simulink model "Laba2_2"  (R2022a)
settings: Solver=VariableStepAuto  StartTime=0.0  StopTime=10.0  RelTol=1e-3
settings Model: Creator=38098  LastModifiedBy=38098

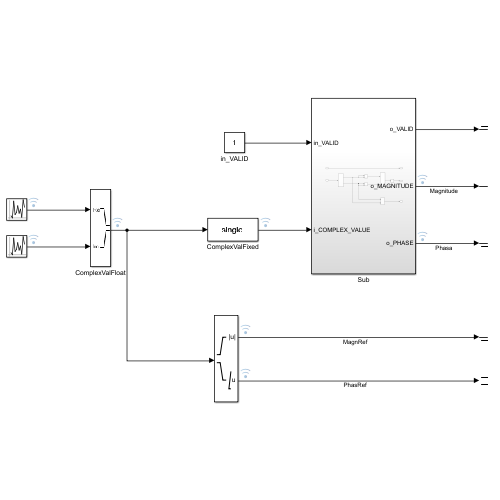
[thumbnail: Simulink's stored preview of the top-level diagram]
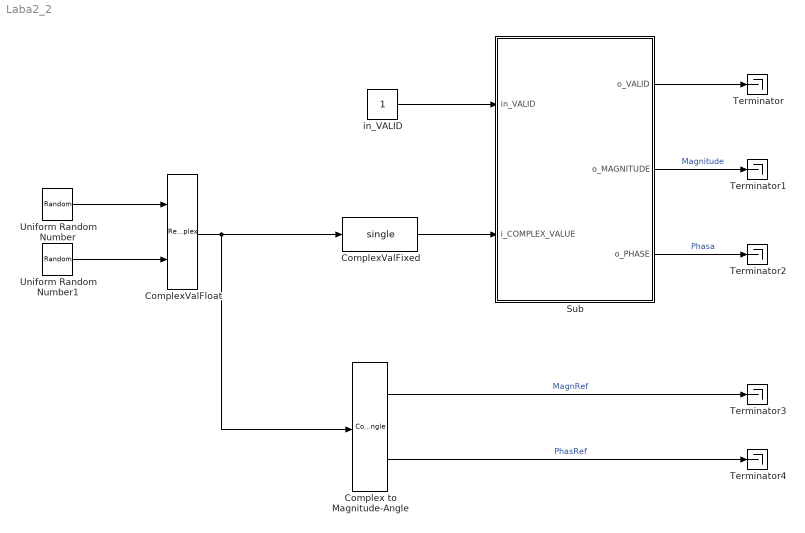
== system Laba2_2 ==
  Complex to Magnitude-Angle : ComplexToMagnitudeAngle
  ComplexValFixed : DataTypeConversion  OutDataTypeStr=single  RndMeth=Round  SaturateOnIntegerOverflow=off
  ComplexValFloat : RealImagToComplex
  Sub : Subsystem
  Terminator{,1..4} (5 alike) : Terminator
  Uniform Random Number : UniformRandomNumber  Minimum=0  Maximum=2 ^(22)-1  Seed=22  SampleTime=1
  Uniform Random Number1 : UniformRandomNumber  Minimum=0  Maximum=2 ^(22)-1  Seed=23  SampleTime=1
  in_VALID : Constant  OutDataTypeStr=boolean  SampleTime=1
  wires:
  Complex to Magnitude-Angle/1 -> Terminator3/1  "MagnRef"
  Sub/1(o_VALID) -> Terminator/1
  Uniform Random Number/1 -> ComplexValFloat/1
  Complex to Magnitude-Angle/2 -> Terminator4/1  "PhasRef"
  in_VALID/1 -> Sub/1(in_VALID)
  Sub/2(o_MAGNITUDE) -> Terminator1/1  "Magnitude"
  ComplexValFloat/1 -> Complex to Magnitude-Angle/1, ComplexValFixed/1
  Uniform Random Number1/1 -> ComplexValFloat/2
  ComplexValFixed/1 -> Sub/2(i_COMPLEX_VALUE)
  Sub/3(o_PHASE) -> Terminator2/1  "Phasa"

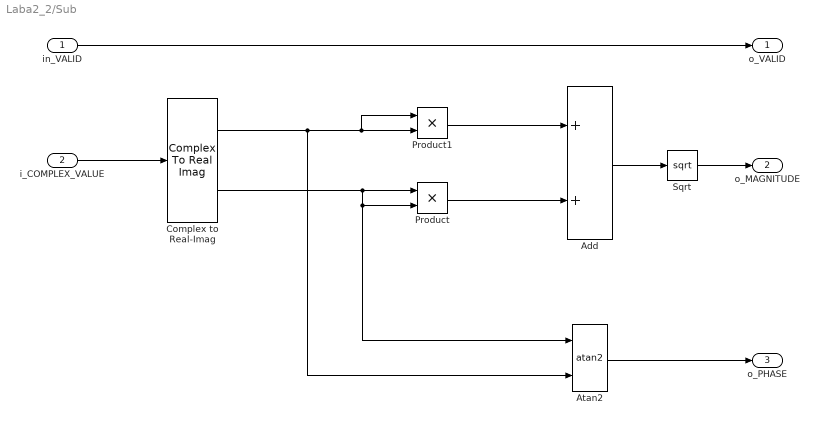
== system Laba2_2/Sub ==
  in_VALID : Inport  OutDataTypeStr=boolean
  i_COMPLEX_VALUE : Inport  Port=2
  Add : Sum
  Atan2 : Trigonometry  Operator=atan2  ApproximationMethod=CORDIC
  Complex to Real-Imag : ComplexToRealImag
  Product : Product
  Product1 : Product
  Sqrt : Sqrt  OutDataTypeStr=Inherit: Inherit via internal rule
  o_VALID : Outport
  o_MAGNITUDE : Outport  Port=2
  o_PHASE : Outport  Port=3
  wires:
  Complex to Real-Imag/1 -> Product1/1, Product1/2, Atan2/2
  Add/1 -> Sqrt/1
  Complex to Real-Imag/2 -> Atan2/1, Product/2, Product/1
  Product1/1 -> Add/1
  Sqrt/1 -> o_MAGNITUDE/1
  Product/1 -> Add/2
  Atan2/1 -> o_PHASE/1
  i_COMPLEX_VALUE/1 -> Complex to Real-Imag/1
  in_VALID/1 -> o_VALID/1
